simulink model "Robot_diferencial"  (R2017b)
settings: Solver=VariableStepAuto  StartTime=0.0  StopTime=Tsim  MinStep=1e-5  RelTol=1e-3
values from neighbouring files (symbols this model uses):
  CI = [0 0 0.3]    [graf.m]
settings Model: Creator=Raúl  LastModifiedBy=Raúl

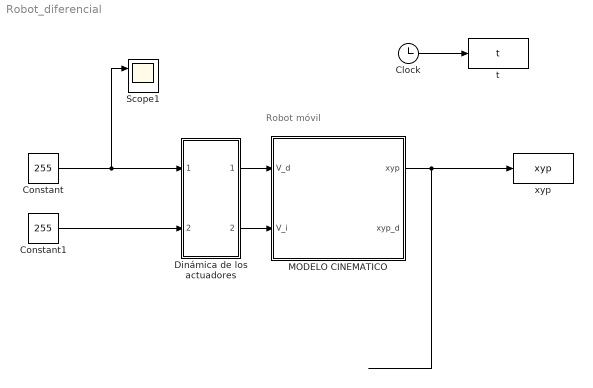
== system Robot_diferencial ==
  note: Robot móvil
  Clock : Clock
  Constant : Constant  Value=255
  Constant1 : Constant  Value=255
  Dinámica de los actuadores : Subsystem
  MODELO CINEMATICO : Subsystem
  Scope1 : Scope  NumInputPorts=2
  t : ToWorkspace  VariableName=t  SampleTime=-1
  xyp : ToWorkspace  VariableName=xyp  SampleTime=-1
  wires:
  MODELO CINEMATICO/1(xyp) -> xyp/1
  Dinámica de los actuadores/1(Out1) -> MODELO CINEMATICO/1(V_d)
  Dinámica de los actuadores/2(Out2) -> MODELO CINEMATICO/2(V_i)
  Clock/1 -> t/1
  Constant/1 -> Scope1/1, Dinámica de los actuadores/1(Vd_ref)
  Constant1/1 -> Dinámica de los actuadores/2(Vi_ref)

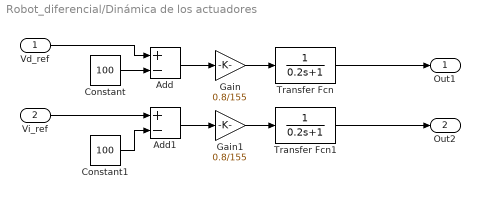
== system Robot_diferencial/Dinámica de los actuadores ==
  Vd_ref : Inport
  Vi_ref : Inport  Port=2
  Add : Sum  Inputs=+-
  Add1 : Sum  Inputs=+-
  Constant : Constant  Value=100
  Constant1 : Constant  Value=100
  Gain : Gain  Gain=0.8/155
  Gain1 : Gain  Gain=0.8/155
  Transfer Fcn : TransferFcn  Denominator=[0.2 1]
  Transfer Fcn1 : TransferFcn  Denominator=[0.2 1]
  Out1 : Outport
  Out2 : Outport  Port=2
  wires:
  Transfer Fcn1/1 -> Out2/1
  Transfer Fcn/1 -> Out1/1
  Gain/1 -> Transfer Fcn/1
  Add/1 -> Gain/1
  Vd_ref/1 -> Add/1
  Constant/1 -> Add/2
  Vi_ref/1 -> Add1/1
  Add1/1 -> Gain1/1
  Gain1/1 -> Transfer Fcn1/1
  Constant1/1 -> Add1/2

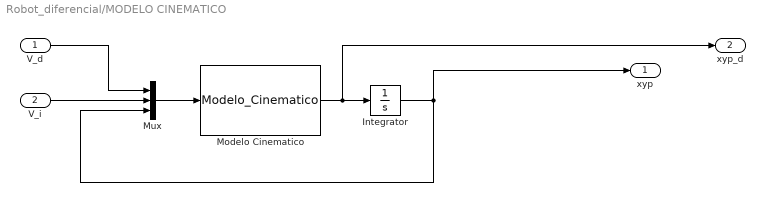
== system Robot_diferencial/MODELO CINEMATICO ==
  V_d : Inport
  V_i : Inport  Port=2
  Integrator : Integrator  InitialCondition=CI
  "Modelo Cinematico " : MATLABFcn  MATLABFcn=Modelo_Cinematico
  Mux : Mux  Inputs=3
  xyp : Outport
  xyp_d : Outport  Port=2
  wires:
  "Modelo Cinematico "/1 -> xyp_d/1, Integrator/1
  V_d/1 -> Mux/1
  Integrator/1 -> xyp/1, Mux/3
  Mux/1 -> "Modelo Cinematico "/1
  V_i/1 -> Mux/2
